simulink model "model41"  (R2024a)
settings: Solver=VariableStepAuto  StartTime=0.0  StopTime=60  RelTol=1e-3
values from neighbouring files (symbols this model uses):
  k = kVal(i)    [script41.m]    (also in script42.m; script43.m)
settings Model: Creator=eva  LastModifiedBy=eva

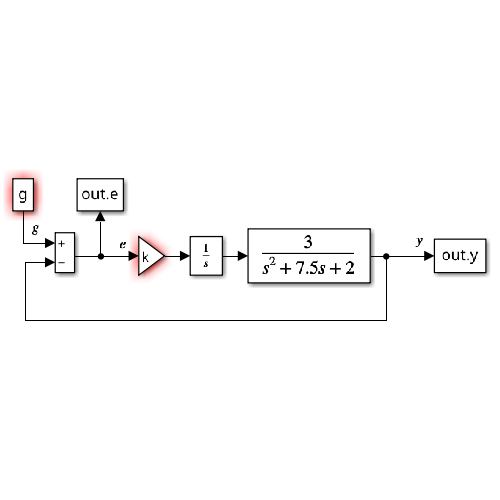
[thumbnail: Simulink's stored preview of the top-level diagram]
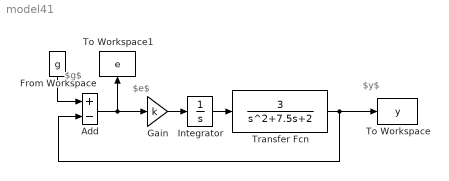
== system model41 ==
  note: $e$
  note: $y$
  note: $g$
  Add : Sum  Inputs=+-
  From Workspace : FromWorkspace  VariableName=g
  Gain : Gain  Gain=k
  Integrator : Integrator
  To Workspace : ToWorkspace  VariableName=y  SaveFormat=Structure With Time  SampleTime=-1
  To Workspace1 : ToWorkspace  VariableName=e  SaveFormat=Structure With Time  SampleTime=-1
  Transfer Fcn : TransferFcn  Numerator=[3]  Denominator=[1 7.5 2]
  wires:
  Add/1 -> To Workspace1/1, Gain/1
  From Workspace/1 -> Add/1
  Gain/1 -> Integrator/1
  Transfer Fcn/1 -> To Workspace/1, Add/2
  Integrator/1 -> Transfer Fcn/1
